simulink model "ArduinoInterface"  (R2024b)
settings: Solver=FixedStepAuto  StartTime=0.0  StopTime=inf  FixedStep=0.0001  RelTol=1e-3  EnableMultiTasking=on
libraries: arduinolib x6, eeGeneralControl x4, simulink x1, arduinosensorlib x1, simulink_extras x1
settings Model: ExtModeTrigDuration=2  Creator=Mario Medhat  LastModifiedBy=Mariam
settings SolverCC: AutoInsertRateTranBlk=on
settings OptimizationCC: EnhancedBackFolding=on  PassReuseOutputArgsAs=Individual arguments  ZeroExternalMemoryAtStartup=off  ZeroInternalMemoryAtStartup=off  MaxStackSize=64  OptimizeBlockOrder=speed  DifferentSizesBufferReuse=on  OptimizationCustomize=off  EfficientTunableParamExpr=on
settings DebuggingCC: ParameterTunabilityLossMsg=error
settings HardwareCC: ProdBitPerInt=16  ProdBitPerPointer=16  ProdBitPerSizeT=16  ProdBitPerPtrDiffT=16  ProdLargestAtomicInteger=Integer  ProdWordSize=8  ProdHWDeviceType=Atmel->AVR
settings SFSimCC: MATLABDynamicMemAlloc=off
settings RTWCC: Description=Embedded Coder  SystemTargetFile=ert.tlc  HardwareBoard=Arduino Uno  TemplateMakefile=ert_default_tmf  Toolchain=Arduino AVR  BuildConfiguration=Faster Runs
settings CodeAppCC: ForceParamTrailComments=on  IgnoreCustomStorageClasses=off  OperatorAnnotations=on  SimulinkDataObjDesc=on  SFDataObjDesc=on  InsertBlockDesc=on
settings ERTTargetCC: SupportContinuousTime=on  SupportVariableSizeSignals=on  ExtModeTransport=3  ExtModeStaticAlloc=on  ExtModeAutomaticAllocSize=off  ExtModeStaticAllocSize=250  ExtModeMexFile=ext_xcp  ExtModeIntrfLevel=Level2 - Open  InlinedParameterPlacement=Hierarchical  DynamicArrayContainerType=coder::array

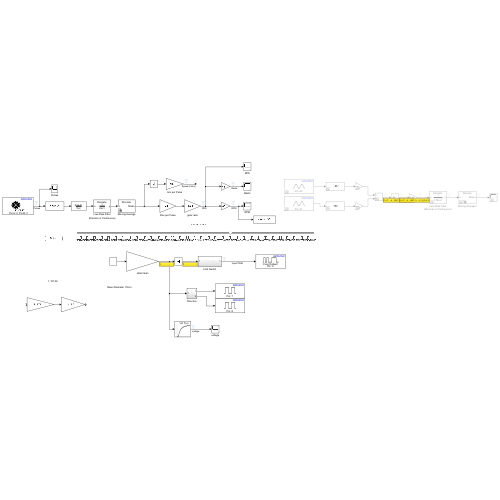
[thumbnail: Simulink's stored preview of the top-level diagram]
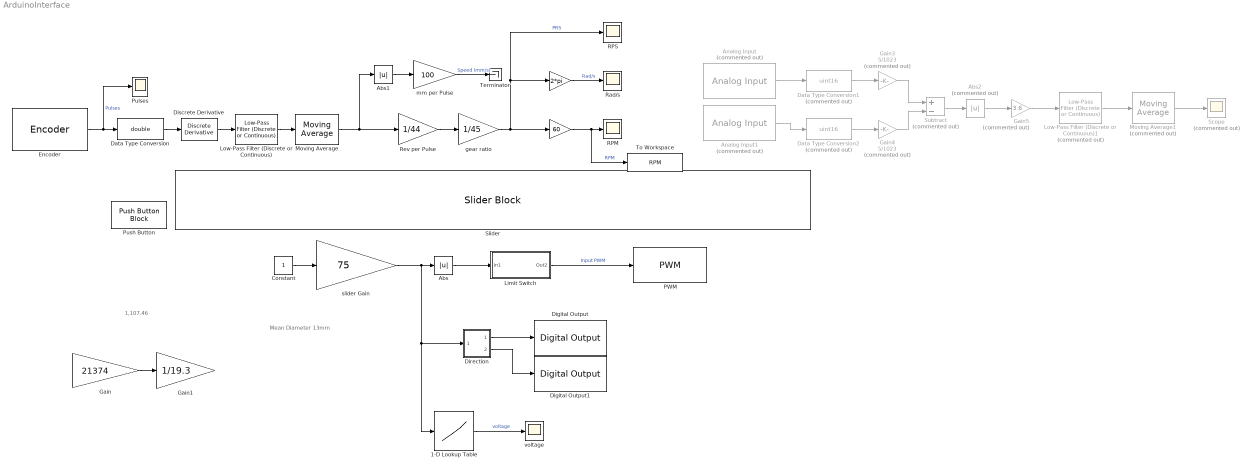
== system ArduinoInterface ==
  note: Mean Diameter 13mm
  note: 1,107.46
  " " : Gain  Gain=60
  "   " : Gain  Gain=2*pi
  1-D Lookup Table : Lookup_n-D  NumberOfTableDimensions=1  BreakpointsForDimension1=[0 5 10 15 20 25 30 35 40 45 50 55 60 65 70 75 80 85 90 95 100 105 110 115 120 125 130 135 140 145 150 155 160 165 170 175 180 185 190 195 200 205 210 215 220 225 230 235 240 245 250 255]  Table=[0;0.01;0.029999999999999999;0.050000000000000003;0.10000000000000001;0.13;0.17999999999999999;0.23000000000000001;2.5;3.0800000000000001;3.77;4.54;5.0800000000000001;5.5499999999999998;6.0499999999999998;6.5;6.9699999999999998;7.2300000000000004;7.5099999999999998;7.7199999999999998;7.9000000000000004;8.0899999999999999;8.2799999999999994;8.4000000000000004;8.5600000000000005;8.6500000000000004;8.8699999999999992;9.3000000000000007;9.2699999999999996;9.3300000000000001;9.4499999999999993;9.5099999999999998;9.5899999999999999;9.6600000000000001;9.7400000000000002;9.8200000000000003;9.8900000000000006;9.9100000000000001;9.9600000000000009;10.039999999999999;10.08;10.109999999999999;10.140000000000001;10.199999999999999;10.26;10.31;10.369999999999999;10.43;10.470000000000001;10.470000000000001;10.52;10.74]  InternalRulePriority=Speed  RndMeth=Simplest
  Abs : Abs  SaturateOnIntegerOverflow=off
  Abs1 : Abs  SaturateOnIntegerOverflow=off
  Abs2 : Abs  Commented=on  SaturateOnIntegerOverflow=off
  Analog Input : arduinolib/Analog Input  Commented=on  pinNumber=0  ReadResultsOnly=off  ConversionTriggerSource=Software  ExternalTriggerType=uint32( 0 )  OutputDataType=uint16  EnableConversionCompleteNotify=off  EnableOuputStatus=off  SampleTime=-1  blockPlatform=arduino
  Analog Input1 : arduinolib/Analog Input  Commented=on  pinNumber=1  ReadResultsOnly=off  ConversionTriggerSource=Software  ExternalTriggerType=uint32( 0 )  OutputDataType=uint16  EnableConversionCompleteNotify=off  EnableOuputStatus=off  SampleTime=-1  blockPlatform=arduino
  Constant : Constant
  Data Type Conversion : DataTypeConversion  OutDataTypeStr=double  SaturateOnIntegerOverflow=off  RndMeth=Floor
  Data Type Conversion1 : DataTypeConversion  Commented=on  OutDataTypeStr=uint16  SaturateOnIntegerOverflow=off  RndMeth=Floor
  Data Type Conversion2 : DataTypeConversion  Commented=on  OutDataTypeStr=uint16  SaturateOnIntegerOverflow=off  RndMeth=Floor
  Digital Output : arduinolib/Digital Output  pinNumber=7  Direction=output  blockPlatform=arduino
  Digital Output1 : arduinolib/Digital Output  pinNumber=8  Direction=output  blockPlatform=arduino
  Direction : Subsystem
  Discrete Derivative : simulink/Discrete/Discrete Derivative  gainval=1.0  ICPrevScaledInput=0.0  OutMin=[]  OutMax=[]  OutDataType=fixdt(1, 16)  OutScaling=2^-10  DoSatur=off
  Encoder : arduinosensorlib/Encoder  InputA=2  InputB=3  Mode=No reset  SampleTime=-1
  Gain : Gain  Gain=21374
  Gain1 : Gain  Gain=1/19.3
  Gain3 : Gain  Commented=on  Gain=5/1023  OutDataTypeStr=double
  Gain4 : Gain  Commented=on  Gain=5/1023  OutDataTypeStr=double
  Gain5 : Gain  Commented=on  Gain=3.6  OutDataTypeStr=double
  Limit Switch : Subsystem
  Low-Pass Filter (Discrete or Continuous) : eeGeneralControl/Low-Pass Filter (Discrete or Continuous)  K=1  T=2  B=inf  A=-inf  init_option=Inherited from block input  x0=0  Ts=-1
  Low-Pass Filter (Discrete or Continuous)1 : eeGeneralControl/Low-Pass Filter (Discrete or Continuous)  Commented=on  K=1  T=1.15  B=inf  A=-inf  init_option=Inherited from block input  x0=0  Ts=-1
  Moving Average : eeGeneralControl/Moving Average  VariantControl=Variant1  LabelModeActiveChoice=Discrete  f=1000  x0=0  BufferSize=8192  Ts=-1
      settings: LibrarySourceBlock=ee_sl_lib/General Control/Moving Average
  Moving Average1 : eeGeneralControl/Moving Average  Commented=on  VariantControl=Variant1  LabelModeActiveChoice=Discrete  f=1  x0=0  BufferSize=8192  Ts=-1
      settings: LibrarySourceBlock=ee_sl_lib/General Control/Moving Average
  PWM : arduinolib/PWM  pinNumber=9  frequencyType=Default  desiredFrequency=490.2  achievableFrequency=490.2
  Pulses : Scope
  Push Button : PushButtonBlock  OffValue=0.000000
  RPM : Scope
  RPS : Scope
  Rad/s : Scope
  Rev per Pulse : Gain  Gain=1/44
  Scope : Scope  Commented=on
  Slider : SliderBlock  ScaleMin=-255  ScaleMax=255  TickInterval=5
  Subtract : Sum  Commented=on  Inputs=+-
  Terminator : Terminator
  To Workspace : ToWorkspace  VariableName=RPM  SaveFormat=Timeseries  SampleTime=-1
  gear ratio : Gain  Gain=1/45
  mm per Pulse : Gain  Gain=100
  slider Gain : Gain  Gain=75  ParamDataTypeStr=int16
  voltage : Scope
  wires:
  Encoder/1 -> Pulses/1, Data Type Conversion/1  "Pulses"
  Data Type Conversion/1 -> Discrete Derivative/1
  Rev per Pulse/1 -> gear ratio/1
  gear ratio/1 -> "   "/1, RPS/1, " "/1  "PRS"
  " "/1 -> To Workspace/1, RPM/1  "RPM"
  "   "/1 -> Rad/s/1  "Rad/s"
  Constant/1 -> slider Gain/1
  Abs/1 -> Limit Switch/1(In1)
  Limit Switch/1(Out2) -> PWM/1  "Input PWM"
  Direction/1(Out1) -> Digital Output/1
  Direction/2(Out2) -> Digital Output1/1
  Gain/1 -> Gain1/1
  mm per Pulse/1 -> Terminator/1  "Speed (mm/s)"
  Abs1/1 -> mm per Pulse/1
  Discrete Derivative/1 -> Low-Pass Filter (Discrete or Continuous)/1
  Low-Pass Filter (Discrete or Continuous)/1 -> Moving Average/1
  Moving Average/1 -> Abs1/1, Rev per Pulse/1
  Analog Input/1 -> Data Type Conversion1/1
  Gain3/1 -> Subtract/1
  Gain4/1 -> Subtract/2
  Subtract/1 -> Abs2/1
  Abs2/1 -> Gain5/1
  Gain5/1 -> Low-Pass Filter (Discrete or Continuous)1/1
  Analog Input1/1 -> Data Type Conversion2/1
  Data Type Conversion1/1 -> Gain3/1
  Data Type Conversion2/1 -> Gain4/1
  Low-Pass Filter (Discrete or Continuous)1/1 -> Moving Average1/1
  Moving Average1/1 -> Scope/1
  slider Gain/1 -> Direction/1(In1), 1-D Lookup Table/1, Abs/1
  1-D Lookup Table/1 -> voltage/1  "voltage"

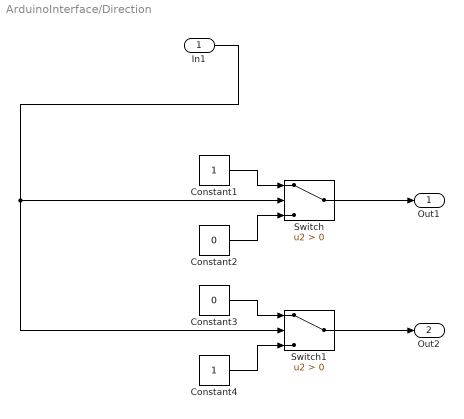
== system ArduinoInterface/Direction ==
  In1 : Inport
  Constant1 : Constant
  Constant2 : Constant  Value=0
  Constant3 : Constant  Value=0
  Constant4 : Constant
  Switch : Switch  Criteria=u2 > Threshold  SaturateOnIntegerOverflow=off  InputSameDT=off
  Switch1 : Switch  Criteria=u2 > Threshold  SaturateOnIntegerOverflow=off  InputSameDT=off
  Out1 : Outport
  Out2 : Outport  Port=2
  wires:
  In1/1 -> Switch1/2, Switch/2
  Constant3/1 -> Switch1/1
  Constant1/1 -> Switch/1
  Constant2/1 -> Switch/3
  Constant4/1 -> Switch1/3
  Switch/1 -> Out1/1
  Switch1/1 -> Out2/1

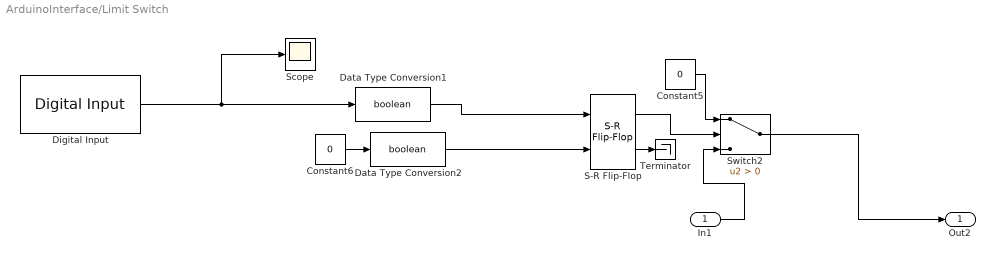
== system ArduinoInterface/Limit Switch ==
  In1 : Inport
  Constant5 : Constant  Value=0
  Constant6 : Constant  Value=0
  Data Type Conversion1 : DataTypeConversion  OutDataTypeStr=boolean  SaturateOnIntegerOverflow=off  RndMeth=Floor
  Data Type Conversion2 : DataTypeConversion  OutDataTypeStr=boolean  SaturateOnIntegerOverflow=off  RndMeth=Floor
  Digital Input : arduinolib/Digital Input  pinNumber=6  mode=Default  Direction=input  SampleTime=0.1  blockPlatform=arduino
  S-R Flip-Flop : simulink_extras/Flip Flops/S-R Flip-Flop  initial_condition=0
  Scope : Scope
  Switch2 : Switch  Criteria=u2 > Threshold  SaturateOnIntegerOverflow=off  InputSameDT=off
  Terminator : Terminator
  Out2 : Outport
  wires:
  Constant6/1 -> Data Type Conversion2/1
  Digital Input/1 -> Scope/1, Data Type Conversion1/1
  Switch2/1 -> Out2/1
  Constant5/1 -> Switch2/1
  S-R Flip-Flop/1 -> Switch2/2
  Data Type Conversion2/1 -> S-R Flip-Flop/2
  S-R Flip-Flop/2 -> Terminator/1
  Data Type Conversion1/1 -> S-R Flip-Flop/1
  In1/1 -> Switch2/3
